simulink model "VDC_2023"  (R2023a)
settings: Solver=FixedStepAuto  StartTime=0.0  StopTime=10.0  RelTol=1e-3
libraries: simulink x4
(part 1 of 2)
settings Model: Creator=no  LastModifiedBy=no
settings OptimizationCC: DefaultParameterBehavior=Inlined
settings RTWCC: Description=INTECRIO Real-Time Target  SystemTargetFile=irt.tlc  TemplateMakefile=irt_default_tmf
settings STFCustomTargetCC: UtilityFuncGeneration=Shared location  ConcurrentExecutionCompliant=off  MatFileLogging=on  UseToolchainInfoCompliant=off  SystemTargetFile=irt.tlc
settings GRTTargetCC: UtilityFuncGeneration=Shared location  ParMdlRefBuildCompliant=off  CompOptLevelCompliant=off  ConcurrentExecutionCompliant=off  CombineOutputUpdateFcns=off  CPPClassGenCompliant=off  GRTInterface=on  UseToolchainInfoCompliant=off  GenerateASAP2=on

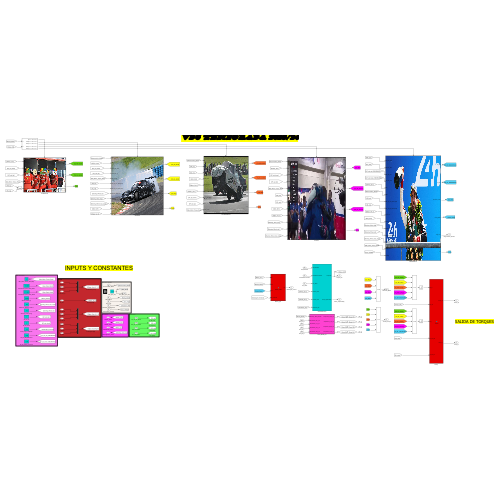
[thumbnail: Simulink's stored preview of the top-level diagram]
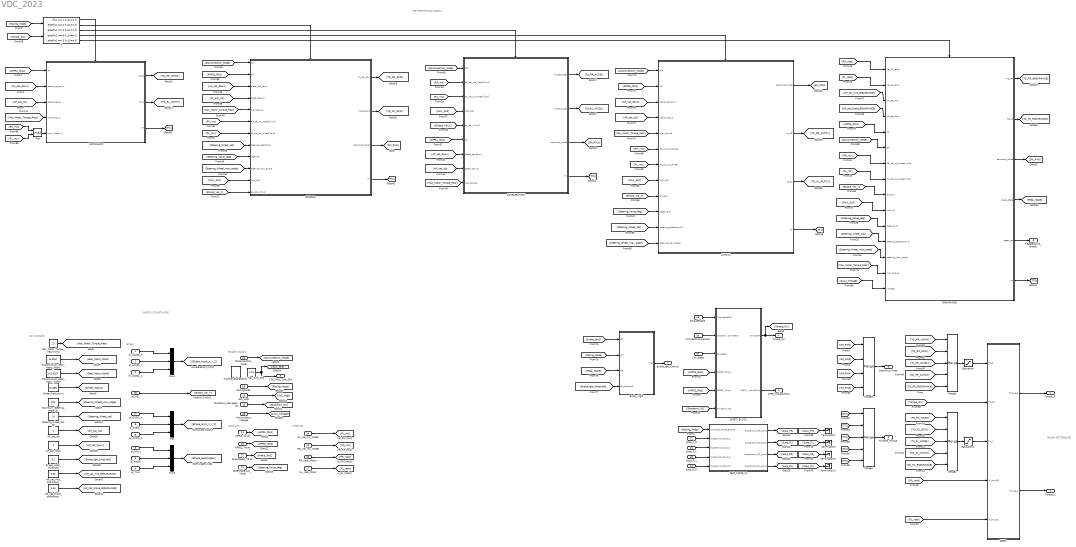
== system VDC_2023 ==
  note: VDC TEMPORADA 2023/24
  note: INPUTS Y CONSTANTES
  note: SALIDA DE TORQUES
  note: Ellipse
  note: Sensorics
  note: Velocities
  note: Car constants
  note: Random Signals
  el_ACCEL_X : Inport
  el_ACCEL_Y : Inport  Port=2
  el_ACCEL_Z : Inport  Port=3
  el_YAW : Inport  Port=4
  el_PITCH : Inport  Port=5
  el_ROLL : Inport  Port=6
  el_GYRO_X : Inport  Port=7
  el_GYRO_Y : Inport  Port=8
  el_GYRO_Z : Inport  Port=9
  APPS2_Value : Inport  Port=10
  APPS1_Value : Inport  Port=11
  BrakePedal_Value : Inport  Port=12
  SteeringSensor_Value : Inport  Port=13
  RL_Vel_ms_Wheel : Inport  Port=14
  RR_Vel_ms_Wheel : Inport  Port=15
  RR_rads_Motor : Inport  Port=16
  RL_rads_Motor : Inport  Port=17
  Accumulator_Voltage : Inport  Port=18
  Shutdown_PackageIntck : Inport  Port=19
  Disconnection_Mode : Inport  Port=20
  Susp_F_L : Inport  Port=21
  Susp_F_R : Inport  Port=22
  Susp_R_L : Inport  Port=23
  Susp_R_R : Inport  Port=24
  TorqueEnable : Inport  Port=25
  CriticalDisconnection : Inport  Port=26
  Car_State : Inport  Port=27
  RacingMode : Inport  Port=28
  SoC_High : Inport  Port=29
  el_VEL : Inport  Port=30
  ACCELERATION : Subsystem
      mask Display: image('flight-simulator-x-4e263b2eefc8e-3478716029.jpg');
  AP_sat_brake_endurance : Constant  Value=0.45
  AP_sat_down : Constant  Value=0
  AP_sat_mid_endurance : Constant  Value=0.55
  AP_sat_up : Constant
  AUTOX1 : Subsystem
      mask Display: image('autox.jpg');
  Brake_Light : MATLAB Function  TreatAsAtomicUnit=on
  Brake_Light_Threshold : Constant  Value=0.2
  ENDURANCE : Subsystem
      mask Display: image('endurance.jpg');
  Function Explanation : simulink/Model-Wide Utilities/DocBlock  DocumentType=Text
      content=|
      | Comparing the speed of the Ellipse and the speed of the Wheels, we can
      | determine the % of deviation between both (which is the slip). With
      | calculations from the Tyres & Performance Department, we know that the
      | maximum optimal slip in a STRAIGHT line is 15%. Therefore (using the Magic
      | Formula), we can determine the maximum X-Force permissible by the Wheels
      | with that % of slip (which is the constant Max_Fx_Tyre, input
      | of Rigid Axle).
      |
      | With that and the radius of the Wheels, we can calculate the maximum
      | Torque for it to stop slipping.
  If : If  NumInputs=2  IfExpression=u1 == 1 & u2 == 1  ElseIfExpressions=u1 == 2 & u2 == 1, u1 == 3 & u2 == 1, u1 == 4 & u2 == 1, u1 == 5 & u2 == 1  ShowElse=off
  Max : MinMax  Function=max  Inputs=2
  Max_Motor_Torque_Rear [Nm] : Constant  Value=27
  Max_Tyre_Slip : Constant  Value=1.15
  Maximum_Steering_angle [º] : Constant  Value=125
  Merge1 : Merge  Inputs=5
  Merge2 : Merge  Inputs=5
  Merge3 : Merge  Inputs=4
  Merge4 : Merge  Inputs=5
  Mux : Mux  Inputs=3
  Mux1 : Mux  Inputs=3
  Mux3 : Mux  Inputs=3
  SAFETY BLOCK : Subsystem
  SKIDPAD : Subsystem
      mask Display: image('MZR_MadMike_Okayama_36_12-4221701208.jpg');
  Safety : MATLAB Function  TreatAsAtomicUnit=on
  Saturation : Saturate  UpperLimit=27  LowerLimit=-27
  Saturation1 : Saturate  UpperLimit=27  LowerLimit=-27
  Steering_wheel_sat [º] : Constant  Value=10
  TEST_MODE_IN : Subsystem  TreatAsAtomicUnit=on
  Terminator{2..3,10..11} (4 alike) : Terminator
  Transmission_Gear_Ratio_MtoW : Constant  Value=11.3257
  Transmission_Gear_Ratio_WtoM : Constant  Value=1/11.3257
  WORKSHOP : Subsystem
      mask Display: image('workshop.jpg');
  Wheel_Radius [m] : Constant  Value=0.2285
  Torque_R : Outport
  Torque_L : Outport  Port=2
  APPS_Implausibility : Outport  Port=3  VectorParamsAs1DForOutWhenUnconnected=off
  Torque_OK : Outport  Port=4  VectorParamsAs1DForOutWhenUnconnected=off
  VDC_Max_Tyre_Slip : Outport  Port=5
  Sensorics_Mode : Outport  Port=6
  BrakeLight_Control : Outport  Port=7  VectorParamsAs1DForOutWhenUnconnected=off
  Regenerative_Enable : Outport  Port=8
  Throttle_Torque : Outport  Port=9
  wires:
  el_PITCH/1 -> Mux3/2
  el_GYRO_Z/1 -> Mux/3
  el_ACCEL_Y/1 -> Mux1/2
  Mux3/1 -> [Ellipse_EulerAngles]
  el_ROLL/1 -> Mux3/1
  Mux1/1 -> [Ellipse_Accel_X_Y_Z]
  el_YAW/1 -> Mux3/3
  el_GYRO_X/1 -> Mux/1
  el_ACCEL_X/1 -> Mux1/1
  Mux/1 -> [Ellipse_Gyro_X_Y_Z]
  el_GYRO_Y/1 -> Mux/2
  el_ACCEL_Z/1 -> Mux1/3
  SteeringSensor_Value/1 -> [Steering_Value_deg]
  APPS1_Value/1 -> [APPS1_0to1]
  BrakePedal_Value/1 -> [Brake_0to1]
  APPS2_Value/1 -> [APPS2_0to1]
  Transmission_Gear_Ratio_MtoW/1 -> [Gear_Ratio_MtoW]
  Transmission_Gear_Ratio_WtoM/1 -> [Gear_Ratio_WtoM]
  Wheel_Radius [m]/1 -> [Wheel_Radius]
  Max_Motor_Torque_Rear [Nm]/1 -> [Max_Motor_Torque_Rear]
  Shutdown_PackageIntck/1 -> [Shutdown_OK]
  Accumulator_Voltage/1 -> [Accu_Voltage]
  Maximum_Steering_angle [º]/1 -> [Steering_Wheel_max_angle]
  Steering_wheel_sat [º]/1 -> [Steering_Wheel_sat]
  Disconnection_Mode/1 -> [Disconnection_Mode]
  TEST_MODE_IN/2(Suspension_FL_N_out) -> [Susp_FL]
  [Racing_Mode] -> TEST_MODE_IN/1(Workshop_Mode_Enable)
  Susp_F_R/1 -> TEST_MODE_IN/2(Suspension_FR_N_in)
  Susp_R_L/1 -> TEST_MODE_IN/4(Suspension_RL_N_in)
  Susp_R_R/1 -> TEST_MODE_IN/5(Suspension_RR_N_in)
  TEST_MODE_IN/3(Suspension_RR_N_out) -> [Susp_RR]
  Susp_F_L/1 -> TEST_MODE_IN/3(Suspension_FL_N_in)
  TEST_MODE_IN/4(Suspension_RL_N_out) -> [Susp_RL]
  TEST_MODE_IN/1(Suspension_FR_N_out) -> [Susp_FR]
  Max_Tyre_Slip/1 -> [MAX_SLR], VDC_Max_Tyre_Slip/1
  CriticalDisconnection/1 -> SAFETY BLOCK/2(CriticalDisconnection)
  TorqueEnable/1 -> SAFETY BLOCK/1(TorqueEnable)
  SAFETY BLOCK/1(TorqueOK) -> Torque_OK/1, [Torque_OK]
  [APPS1_0to1] -> SAFETY BLOCK/4(APPS1_Value)
  SAFETY BLOCK/2(APPS_Implausibility) -> APPS_Implausibility/1
  [APPS2_0to1] -> SAFETY BLOCK/5(APPS2_Value)
  [Shutdown_OK] -> SAFETY BLOCK/6(Shutdown_OK)
  Car_State/1 -> SAFETY BLOCK/3(Car_State)
  AP_sat_up/1 -> [AP_sat_Up]
  AP_sat_down/1 -> [AP_sat_down]
  [Susp_FL] -> Terminator3/1
  [Susp_RL] -> Terminator11/1
  [Susp_RR] -> Terminator10/1
  [Susp_FR] -> Terminator2/1
  [Tq_RR_ACCEL] -> Merge2/3
  [TQ_RR_AUTOX] -> Merge2/4
  [TQ_RR_WORK] -> Merge2/1
  [TQ_RR_SKID] -> Merge2/2
  RacingMode/1 -> [Racing_Mode]
  [APPS1_0to1] -> WORKSHOP/1(AP)
  [AP_sat_down] -> WORKSHOP/2(pedal_sat_down)
  [AP_sat_Up] -> WORKSHOP/3(pedal_sat_up)
  [Max_Motor_Torque_Rear] -> WORKSHOP/4(max_torque)
  [TQ_RR_ENDURANCE] -> Merge2/5
  [TQ_RL_ENDURANCE] -> Merge1/5
  [TQ_RL_SKID] -> Merge1/2
  [TQ_RL_AUTOX] -> Merge1/4
  [Tq_RL_ACCEL] -> Merge1/3
  [TQ_RL_WORK] -> Merge1/1
  WORKSHOP/1(TQ_R) -> [TQ_RR_WORK]
  WORKSHOP/2(TQ_L) -> [TQ_RL_WORK]
  ENDURANCE/2(TQ_RL) -> [TQ_RL_ENDURANCE]
  ENDURANCE/1(TQ_RR) -> [TQ_RR_ENDURANCE]
  [Racing_Mode] -> If/1
  If/1 -> WORKSHOP/Action
  If/2 -> SKIDPAD/Action
  If/3 -> ACCELERATION/Action
  If/4 -> AUTOX1/Action
  If/5 -> ENDURANCE/Action
  [MAX_SLR] -> ENDURANCE/10(max_slr)
  [Disconnection_Mode] -> ENDURANCE/6(DM)
  RL_rads_Motor/1 -> [RL_rads]
  RR_rads_Motor/1 -> [RR_rads]
  RR_Vel_ms_Wheel/1 -> [RR_ms]
  RL_Vel_ms_Wheel/1 -> [RL_ms]
  [RR_rads] -> ENDURANCE/1(Vel_RR_rad/s)
  [RL_rads] -> ENDURANCE/2(Vel_RL_rad/s)
  [RR_ms] -> ENDURANCE/7(RR_Vel_ms_Wheel [m/s])
  [RL_ms] -> ENDURANCE/8(RL_Vel_ms_Wheel [m/s])
  [Steering_Wheel_sat] -> ENDURANCE/12(steering_deadzone (º))
  [Steering_Value_deg] -> ENDURANCE/11(steering (º))
  [Steering_Wheel_max_angle] -> ENDURANCE/13(steering_max_angle)
  [APPS1_0to1] -> ENDURANCE/5(AP)
  SoC_High/1 -> [SoC_High]
  ACCELERATION/1(Tq_RR_accel) -> [Tq_RR_ACCEL]
  ACCELERATION/2(Tq_RL_accel) -> [Tq_RL_ACCEL]
  SKIDPAD/1(Tq_RR_Skid) -> [TQ_RR_SKID]
  SKIDPAD/2(Tq_RL_Skid) -> [TQ_RL_SKID]
  [Disconnection_Mode] -> SKIDPAD/1(DM)
  [Disconnection_Mode] -> ACCELERATION/1(DM)
  [RR_ms] -> SKIDPAD/6(RR_Vel_ms_Wheel [m/s])
  [RL_ms] -> SKIDPAD/7(RL_Vel_ms_Wheel [m/s])
  [RL_ms] -> ACCELERATION/3(RL_Vel_ms_Wheel [m/s])
  [RR_ms] -> ACCELERATION/2(RR_Vel_ms_Wheel [m/s])
  [APPS1_0to1] -> SKIDPAD/2(AP)
  [Steering_Value_deg] -> SKIDPAD/9(steering)
  [APPS1_0to1] -> ACCELERATION/6(AP)
  [AP_sat_down] -> SKIDPAD/3(pedal_sat_down)
  [AP_sat_Up] -> SKIDPAD/4(pedal_sat_up)
  [AP_sat_down] -> ACCELERATION/7(pedal_sat_down)
  [AP_sat_Up] -> ACCELERATION/8(pedal_sat_up)
  [Max_Motor_Torque_Rear] -> SKIDPAD/5(max_torque)
  [Max_Motor_Torque_Rear] -> ACCELERATION/9(max_torque)
  [MAX_SLR] -> SKIDPAD/11(MAX_SLR)
  [Steering_Wheel_sat] -> SKIDPAD/8(steering_deadzone)
  [Steering_Wheel_max_angle] -> SKIDPAD/10(steering_max_angle)
  [MAX_SLR] -> ACCELERATION/4(MAX_SLR)
  [Torque_OK] -> If/2
  Merge3/1 -> Sensorics_Mode/1
  [SM_RM2] -> Merge3/1
  [SM_RM4] -> Merge3/3
  [SM_RM5] -> Merge3/4
  [SM_RM3] -> Merge3/2
  SKIDPAD/3(sensorics_mode) -> [SM_RM2]
  ACCELERATION/3(sensorics_mode) -> [SM_RM3]
  ENDURANCE/3(sensorics_mode) -> [SM_RM5]
  AUTOX1/1(sensorics_mode) -> [SM_RM4]
  AUTOX1/2(tq_RR) -> [TQ_RR_AUTOX]
  AUTOX1/3(tq_RL) -> [TQ_RL_AUTOX]
  [Steering_Wheel_max_angle] -> AUTOX1/12(steering_max_angle)
  [Steering_Value_deg] -> AUTOX1/10(steering (º))
  [Steering_Wheel_sat] -> AUTOX1/11(steering_deadzone (º))
  [MAX_SLR] -> AUTOX1/8(MAX_SLR)
  [RR_ms] -> AUTOX1/6(RR_vel_ms_Wheel)
  [RL_ms] -> AUTOX1/7(RL_vel_ms_Wheel)
  [Max_Motor_Torque_Rear] -> AUTOX1/5(max_torque)
  [Disconnection_Mode] -> AUTOX1/1(DM)
  [APPS1_0to1] -> AUTOX1/2(AP)
  [AP_sat_down] -> AUTOX1/3(pedal_sat_down)
  [AP_sat_Up] -> AUTOX1/4(pedal_sat_up)
  ENDURANCE/4(Pedal_State) -> [Pedal_State]
  Brake_Light_Threshold/1 -> [BrakeLight_threshold]
  Brake_Light/1(BL) -> BrakeLight_Control/1
  [Brake_0to1] -> Brake_Light/1(BP)
  [Racing_Mode] -> Brake_Light/2(RM)
  [BrakeLight_threshold] -> Brake_Light/4(BL_threshold)
  [Pedal_State] -> Brake_Light/3(PS)
  [Max_Motor_Torque_Rear] -> ENDURANCE/14(max_torque)
  Merge2/1 -> Saturation/1
  Saturation/1 -> Safety/1(Tq_R)
  Merge1/1 -> Saturation1/1
  ENDURANCE/5(regen_en) -> Regenerative_Enable/1
  [Accu_Voltage] -> ENDURANCE/15(voltage)
  WORKSHOP/3(TT) -> [TT1]
  SKIDPAD/4(TT) -> [TT2]
  ACCELERATION/4(TT) -> [TT3]
  AUTOX1/4(TT) -> [TT4]
  ENDURANCE/6(TT) -> [TT5]
  Merge4/1 -> Throttle_Torque/1
  [TT1] -> Merge4/1
  [TT2] -> Merge4/2
  [TT3] -> Merge4/3
  [TT4] -> Merge4/4
  [TT5] -> Merge4/5
  Saturation1/1 -> Safety/3(Tq_L)
  Safety/2(Torque_L) -> Torque_L/1
  Safety/1(Torque_R) -> Torque_R/1
  [Torque_OK] -> Safety/2(Tq_OK)
  [RR_rads] -> Safety/4(W_mot_RR)
  [RL_rads] -> Safety/5(W_mot_RL)
  Max/1 -> WORKSHOP/5(max_wheel_w)
  [RR_ms] -> Max/1
  [RL_ms] -> Max/2
  AP_sat_mid_endurance/1 -> [AP_sat_mid_ENDURANCE]
  AP_sat_brake_endurance/1 -> [AP_sat_brake_ENDURANCE]
  [AP_sat_mid_ENDURANCE] -> ENDURANCE/3(AP_sat_mid)
  [AP_sat_brake_ENDURANCE] -> ENDURANCE/4(AP_sat_down)
  el_VEL/1 -> [Ellipse_Vel_X]
  [Ellipse_Vel_X] -> SKIDPAD/12(el_Vel_X [m/s])
  [Ellipse_Vel_X] -> ACCELERATION/5(el_Vel_X [m/s])
  [Ellipse_Vel_X] -> AUTOX1/9(el_vel_x)
  [Ellipse_Vel_X] -> ENDURANCE/9(el_Vel_X)

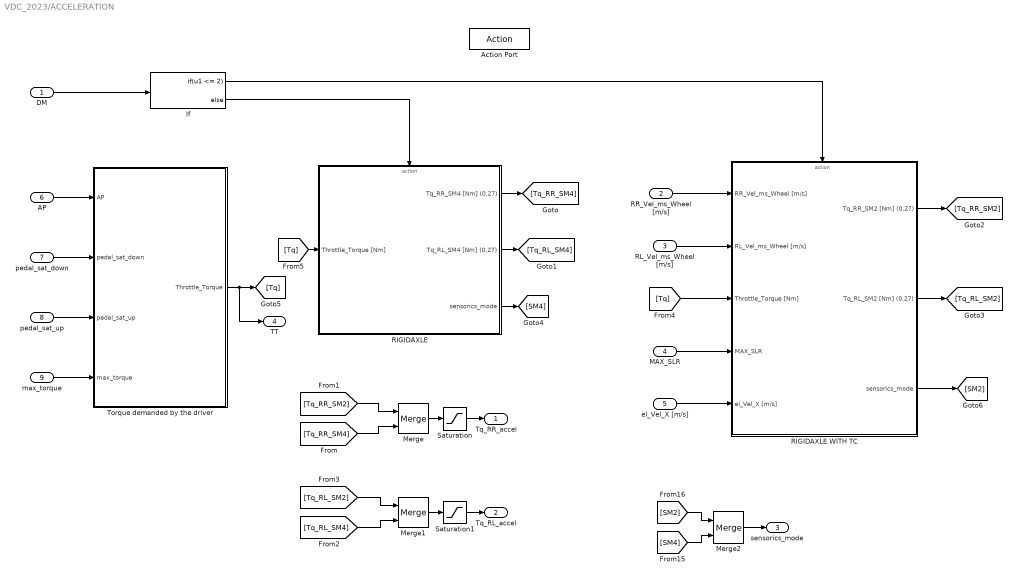
== system VDC_2023/ACCELERATION ==
  DM : Inport
  RR_Vel_ms_Wheel [m/s] : Inport  Port=2
  RL_Vel_ms_Wheel [m/s] : Inport  Port=3
  MAX_SLR : Inport  Port=4
  el_Vel_X [m/s] : Inport  Port=5
  AP : Inport  Port=6
  pedal_sat_down : Inport  Port=7
  pedal_sat_up : Inport  Port=8
  max_torque : Inport  Port=9
  Action Port : ActionPort  ActionPortLabel=elseif( u1 == 3 & u2 == 1)
  If : If  IfExpression=u1 <= 2
  Merge : Merge
  Merge1 : Merge
  Merge2 : Merge
  RIGIDAXLE : Subsystem
  RIGIDAXLE WITH TC : Subsystem
  Saturation : Saturate  UpperLimit=27  LowerLimit=0
  Saturation1 : Saturate  UpperLimit=27  LowerLimit=0
  Torque demanded by the driver : MATLAB Function  TreatAsAtomicUnit=on
  Tq_RR_accel : Outport
  Tq_RL_accel : Outport  Port=2
  sensorics_mode : Outport  Port=3
  TT : Outport  Port=4
  wires:
  DM/1 -> If/1
  If/2 -> RIGIDAXLE/Action
  el_Vel_X [m/s]/1 -> RIGIDAXLE WITH TC/5(el_Vel_X [m/s])
  MAX_SLR/1 -> RIGIDAXLE WITH TC/4(MAX_SLR)
  RL_Vel_ms_Wheel [m/s]/1 -> RIGIDAXLE WITH TC/2(RL_Vel_ms_Wheel [m/s])
  RR_Vel_ms_Wheel [m/s]/1 -> RIGIDAXLE WITH TC/1(RR_Vel_ms_Wheel [m/s])
  AP/1 -> Torque demanded by the driver/1(AP)
  pedal_sat_down/1 -> Torque demanded by the driver/2(pedal_sat_down)
  pedal_sat_up/1 -> Torque demanded by the driver/3(pedal_sat_up)
  max_torque/1 -> Torque demanded by the driver/4(max_torque)
  RIGIDAXLE/1(Tq_RR_SM4 [Nm] (0,27)) -> [Tq_RR_SM4]
  RIGIDAXLE/2(Tq_RL_SM4 [Nm] (0,27)) -> [Tq_RL_SM4]
  RIGIDAXLE WITH TC/2(Tq_RL_SM2 [Nm] (0,27)) -> [Tq_RL_SM2]
  RIGIDAXLE WITH TC/1(Tq_RR_SM2 [Nm] (0,27)) -> [Tq_RR_SM2]
  [Tq_RR_SM4] -> Merge/2
  [Tq_RR_SM2] -> Merge/1
  [Tq_RL_SM4] -> Merge1/2
  [Tq_RL_SM2] -> Merge1/1
  Merge2/1 -> sensorics_mode/1
  [SM4] -> Merge2/2
  [SM2] -> Merge2/1
  RIGIDAXLE/3(sensorics_mode) -> [SM4]
  Torque demanded by the driver/1(Throttle_Torque) -> TT/1, [Tq]
  [Tq] -> RIGIDAXLE WITH TC/3(Throttle_Torque [Nm])
  [Tq] -> RIGIDAXLE/1(Throttle_Torque [Nm])
  RIGIDAXLE WITH TC/3(sensorics_mode) -> [SM2]
  If/1 -> RIGIDAXLE WITH TC/Action
  Merge/1 -> Saturation/1
  Saturation/1 -> Tq_RR_accel/1
  Merge1/1 -> Saturation1/1
  Saturation1/1 -> Tq_RL_accel/1

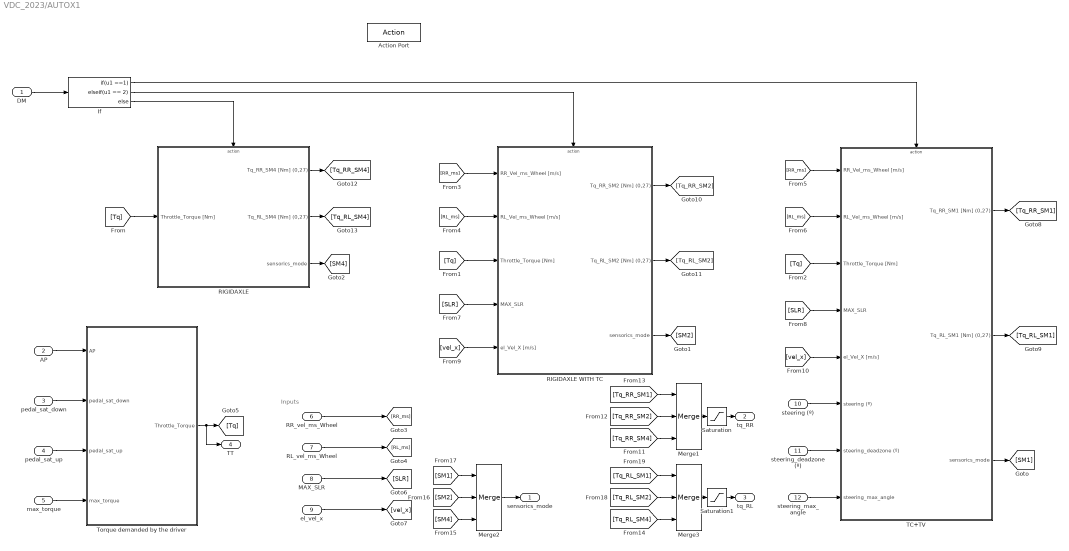
== system VDC_2023/AUTOX1 ==
  note: Inputs
  DM : Inport
  AP : Inport  Port=2
  pedal_sat_down : Inport  Port=3
  pedal_sat_up : Inport  Port=4
  max_torque : Inport  Port=5
  RR_vel_ms_Wheel : Inport  Port=6
  RL_vel_ms_Wheel : Inport  Port=7
  MAX_SLR : Inport  Port=8
  el_vel_x : Inport  Port=9
  steering (º) : Inport  Port=10
  steering_deadzone (º) : Inport  Port=11
  steering_max_angle : Inport  Port=12
  Action Port : ActionPort  ActionPortLabel=elseif( u1 == 4 & u2 == 1)
  If : If  IfExpression=u1 ==1  ElseIfExpressions=u1 == 2
  Merge1 : Merge  Inputs=3
  Merge2 : Merge  Inputs=3
  Merge3 : Merge  Inputs=3
  RIGIDAXLE : Subsystem
  RIGIDAXLE WITH TC : Subsystem
  Saturation : Saturate  UpperLimit=27  LowerLimit=0
  Saturation1 : Saturate  UpperLimit=27  LowerLimit=0
  TC+TV : Subsystem
  Torque demanded by the driver : MATLAB Function  TreatAsAtomicUnit=on
  sensorics_mode : Outport
  tq_RR : Outport  Port=2
  tq_RL : Outport  Port=3
  TT : Outport  Port=4
  wires:
  RIGIDAXLE WITH TC/3(sensorics_mode) -> [SM2]
  TC+TV/3(sensorics_mode) -> [SM1]
  RIGIDAXLE/3(sensorics_mode) -> [SM4]
  [SM2] -> Merge2/2
  [SM4] -> Merge2/3
  Merge2/1 -> sensorics_mode/1
  [SM1] -> Merge2/1
  If/1 -> TC+TV/Action
  If/2 -> RIGIDAXLE WITH TC/Action
  If/3 -> RIGIDAXLE/Action
  DM/1 -> If/1
  pedal_sat_down/1 -> Torque demanded by the driver/2(pedal_sat_down)
  Torque demanded by the driver/1(Throttle_Torque) -> TT/1, [Tq]
  max_torque/1 -> Torque demanded by the driver/4(max_torque)
  pedal_sat_up/1 -> Torque demanded by the driver/3(pedal_sat_up)
  AP/1 -> Torque demanded by the driver/1(AP)
  [Tq] -> RIGIDAXLE/1(Throttle_Torque [Nm])
  [Tq] -> RIGIDAXLE WITH TC/3(Throttle_Torque [Nm])
  [Tq] -> TC+TV/3(Throttle_Torque [Nm])
  RR_vel_ms_Wheel/1 -> [RR_ms]
  RL_vel_ms_Wheel/1 -> [RL_ms]
  [RR_ms] -> RIGIDAXLE WITH TC/1(RR_Vel_ms_Wheel [m/s])
  [RL_ms] -> RIGIDAXLE WITH TC/2(RL_Vel_ms_Wheel [m/s])
  [RR_ms] -> TC+TV/1(RR_Vel_ms_Wheel [m/s])
  [RL_ms] -> TC+TV/2(RL_Vel_ms_Wheel [m/s])
  MAX_SLR/1 -> [SLR]
  el_vel_x/1 -> [vel_x]
  [SLR] -> RIGIDAXLE WITH TC/4(MAX_SLR)
  [SLR] -> TC+TV/4(MAX_SLR)
  [vel_x] -> RIGIDAXLE WITH TC/5(el_Vel_X [m/s])
  [vel_x] -> TC+TV/5(el_Vel_X [m/s])
  steering (º)/1 -> TC+TV/6(steering (º))
  steering_deadzone (º)/1 -> TC+TV/7(steering_deadzone (º))
  steering_max_angle/1 -> TC+TV/8(steering_max_angle)
  [Tq_RR_SM4] -> Merge1/3
  [Tq_RR_SM1] -> Merge1/1
  [Tq_RR_SM2] -> Merge1/2
  [Tq_RL_SM4] -> Merge3/3
  [Tq_RL_SM1] -> Merge3/1
  [Tq_RL_SM2] -> Merge3/2
  TC+TV/1(Tq_RR_SM1 [Nm] (0,27)) -> [Tq_RR_SM1]
  TC+TV/2(Tq_RL_SM1 [Nm] (0,27)) -> [Tq_RL_SM1]
  RIGIDAXLE WITH TC/1(Tq_RR_SM2 [Nm] (0,27)) -> [Tq_RR_SM2]
  RIGIDAXLE WITH TC/2(Tq_RL_SM2 [Nm] (0,27)) -> [Tq_RL_SM2]
  RIGIDAXLE/2(Tq_RL_SM4 [Nm] (0,27)) -> [Tq_RL_SM4]
  RIGIDAXLE/1(Tq_RR_SM4 [Nm] (0,27)) -> [Tq_RR_SM4]
  Merge1/1 -> Saturation/1
  Saturation/1 -> tq_RR/1
  Merge3/1 -> Saturation1/1
  Saturation1/1 -> tq_RL/1

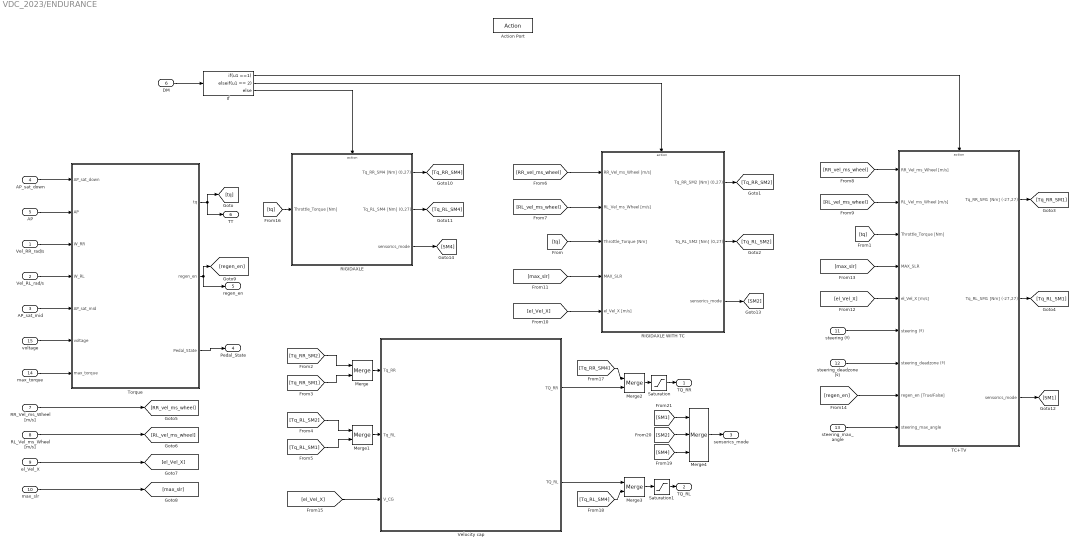
== system VDC_2023/ENDURANCE ==
  Vel_RR_rad/s : Inport
  Vel_RL_rad/s : Inport  Port=2
  AP_sat_mid : Inport  Port=3
  AP_sat_down : Inport  Port=4
  AP : Inport  Port=5
  DM : Inport  Port=6
  RR_Vel_ms_Wheel [m/s] : Inport  Port=7
  RL_Vel_ms_Wheel [m/s] : Inport  Port=8
  el_Vel_X : Inport  Port=9
  max_slr : Inport  Port=10
  steering (º) : Inport  Port=11
  steering_deadzone (º) : Inport  Port=12
  steering_max_angle : Inport  Port=13
  max_torque : Inport  Port=14
  voltage : Inport  Port=15
  Action Port : ActionPort  ActionPortLabel=elseif( u1 == 5 & u2 == 1)
  If : If  IfExpression=u1 ==1  ElseIfExpressions=u1 == 2
  Merge{,1..3} (4 alike) : Merge
  Merge4 : Merge  Inputs=3
  RIGIDAXLE : Subsystem
  RIGIDAXLE WITH TC : Subsystem
  Saturation : Saturate  UpperLimit=27  LowerLimit=-27
  Saturation1 : Saturate  UpperLimit=27  LowerLimit=-27
  TC+TV : Subsystem
  Torque : Subsystem
  Velocity cap : Subsystem
      mask Display: image('iStock-173100947-1675497781.jpg');
  TQ_RR : Outport
  TQ_RL : Outport  Port=2
  sensorics_mode : Outport  Port=3
  Pedal_State : Outport  Port=4
  regen_en : Outport  Port=5
  TT : Outport  Port=6
  wires:
  [tq] -> RIGIDAXLE WITH TC/3(Throttle_Torque [Nm])
  [tq] -> TC+TV/3(Throttle_Torque [Nm])
  RIGIDAXLE WITH TC/1(Tq_RR_SM2 [Nm] (0,27)) -> [Tq_RR_SM2]
  RIGIDAXLE WITH TC/2(Tq_RL_SM2 [Nm] (0,27)) -> [Tq_RL_SM2]
  [Tq_RR_SM2] -> Merge/1
  [Tq_RR_SM1] -> Merge/2
  [Tq_RL_SM2] -> Merge1/1
  [Tq_RL_SM1] -> Merge1/2
  TC+TV/1(Tq_RR_SM1 [Nm] (-27,27)) -> [Tq_RR_SM1]
  TC+TV/2(Tq_RL_SM1 [Nm] (-27,27)) -> [Tq_RL_SM1]
  Merge/1 -> Velocity cap/1(Tq_RR)
  Merge1/1 -> Velocity cap/2(Tq_RL)
  Vel_RR_rad/s/1 -> Torque/3(W_RR)
  Vel_RL_rad/s/1 -> Torque/4(W_RL)
  AP_sat_mid/1 -> Torque/5(AP_sat_mid)
  AP_sat_down/1 -> Torque/1(AP_sat_down)
  AP/1 -> Torque/2(AP)
  DM/1 -> If/1
  RR_Vel_ms_Wheel [m/s]/1 -> [RR_vel_ms_wheel]
  [RR_vel_ms_wheel] -> RIGIDAXLE WITH TC/1(RR_Vel_ms_Wheel [m/s])
  RL_Vel_ms_Wheel [m/s]/1 -> [RL_vel_ms_wheel]
  [RL_vel_ms_wheel] -> RIGIDAXLE WITH TC/2(RL_Vel_ms_Wheel [m/s])
  [RR_vel_ms_wheel] -> TC+TV/1(RR_Vel_ms_Wheel [m/s])
  [RL_vel_ms_wheel] -> TC+TV/2(RL_Vel_ms_Wheel [m/s])
  el_Vel_X/1 -> [el_Vel_X]
  [el_Vel_X] -> RIGIDAXLE WITH TC/5(el_Vel_X [m/s])
  max_slr/1 -> [max_slr]
  [max_slr] -> RIGIDAXLE WITH TC/4(MAX_SLR)
  [el_Vel_X] -> TC+TV/5(el_Vel_X [m/s])
  [max_slr] -> TC+TV/4(MAX_SLR)
  steering (º)/1 -> TC+TV/6(steering (º))
  steering_deadzone (º)/1 -> TC+TV/7(steering_deadzone (º))
  Torque/2(regen_en) -> [regen_en], regen_en/1
  [regen_en] -> TC+TV/8(regen_en [True/False])
  steering_max_angle/1 -> TC+TV/9(steering_max_angle)
  [el_Vel_X] -> Velocity cap/3(V_CG)
  If/2 -> RIGIDAXLE WITH TC/Action
  If/1 -> TC+TV/Action
  [tq] -> RIGIDAXLE/1(Throttle_Torque [Nm])
  RIGIDAXLE/1(Tq_RR_SM4 [Nm] (0,27)) -> [Tq_RR_SM4]
  RIGIDAXLE/2(Tq_RL_SM4 [Nm] (0,27)) -> [Tq_RL_SM4]
  Velocity cap/1(TQ_RR) -> Merge2/2
  [Tq_RR_SM4] -> Merge2/1
  Velocity cap/2(TQ_RL) -> Merge3/1
  [Tq_RL_SM4] -> Merge3/2
  If/3 -> RIGIDAXLE/Action
  [SM1] -> Merge4/1
  Merge4/1 -> sensorics_mode/1
  [SM4] -> Merge4/3
  [SM2] -> Merge4/2
  TC+TV/3(sensorics_mode) -> [SM1]
  RIGIDAXLE WITH TC/3(sensorics_mode) -> [SM2]
  RIGIDAXLE/3(sensorics_mode) -> [SM4]
  Torque/3(Pedal_State) -> Pedal_State/1
  max_torque/1 -> Torque/7(max_torque)
  voltage/1 -> Torque/6(voltage)
  Merge2/1 -> Saturation/1
  Saturation/1 -> TQ_RR/1
  Merge3/1 -> Saturation1/1
  Saturation1/1 -> TQ_RL/1
  Torque/1(tq) -> [tq], TT/1

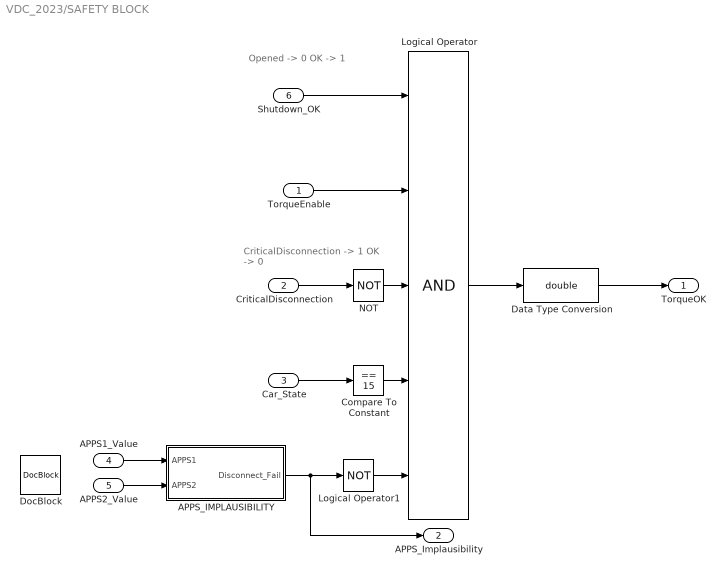
== system VDC_2023/SAFETY BLOCK ==
  note: CriticalDisconnection -> 1
      | OK -> 0
  note: Opened -> 0
      | OK -> 1
  TorqueEnable : Inport
  CriticalDisconnection : Inport  Port=2
  Car_State : Inport  Port=3
  APPS1_Value : Inport  Port=4
  APPS2_Value : Inport  Port=5
  Shutdown_OK : Inport  Port=6
  APPS_IMPLAUSIBILITY : Subsystem
  Compare To Constant : simulink/Logic and Bit Operations/Compare To Constant  relop===  const=15  OutDataTypeStr=boolean
  Data Type Conversion : DataTypeConversion  OutDataTypeStr=double  SaturateOnIntegerOverflow=off  RndMeth=Floor
  DocBlock : simulink/Model-Wide Utilities/DocBlock  DocumentType=Text
      content=|
      | Formula Student Rules 2024 -> T11.8.8
      |     If an implausibility occurs between the values of the APPSs and
      |     persists for more than 100 ms:
      |     • [EV ONLY] The power to the motor(s) must be immediately shut down
      |     completely. It is not necessary to completely deactivate the TS, the
      |     motor controller(s) shutting down the power to the motor(s) is
      |     sufficient.
      |
      | The 'Number_of_Periods' constant, if there's an Implausability, outputs the error X
      | periods (100ms) after the Implausibility happened (25ms * X = 100ms).
  Logical Operator : Logic  Inputs=5  OutDataTypeStr=boolean
  Logical Operator1 : Logic  Operator=NOT  IconShape=distinctive  AllPortsSameDT=off  OutDataTypeStr=boolean
  NOT : Logic  Operator=NOT  IconShape=distinctive  AllPortsSameDT=off  OutDataTypeStr=boolean
  TorqueOK : Outport  VectorParamsAs1DForOutWhenUnconnected=off
  APPS_Implausibility : Outport  Port=2  VectorParamsAs1DForOutWhenUnconnected=off
  wires:
  Logical Operator/1 -> Data Type Conversion/1
  Car_State/1 -> Compare To Constant/1
  NOT/1 -> Logical Operator/3
  CriticalDisconnection/1 -> NOT/1
  TorqueEnable/1 -> Logical Operator/2
  APPS2_Value/1 -> APPS_IMPLAUSIBILITY/2(APPS2)
  APPS1_Value/1 -> APPS_IMPLAUSIBILITY/1(APPS1)
  APPS_IMPLAUSIBILITY/1(Disconnect_Fail) -> APPS_Implausibility/1, Logical Operator1/1
  Compare To Constant/1 -> Logical Operator/4
  Shutdown_OK/1 -> Logical Operator/1
  Logical Operator1/1 -> Logical Operator/5
  Data Type Conversion/1 -> TorqueOK/1

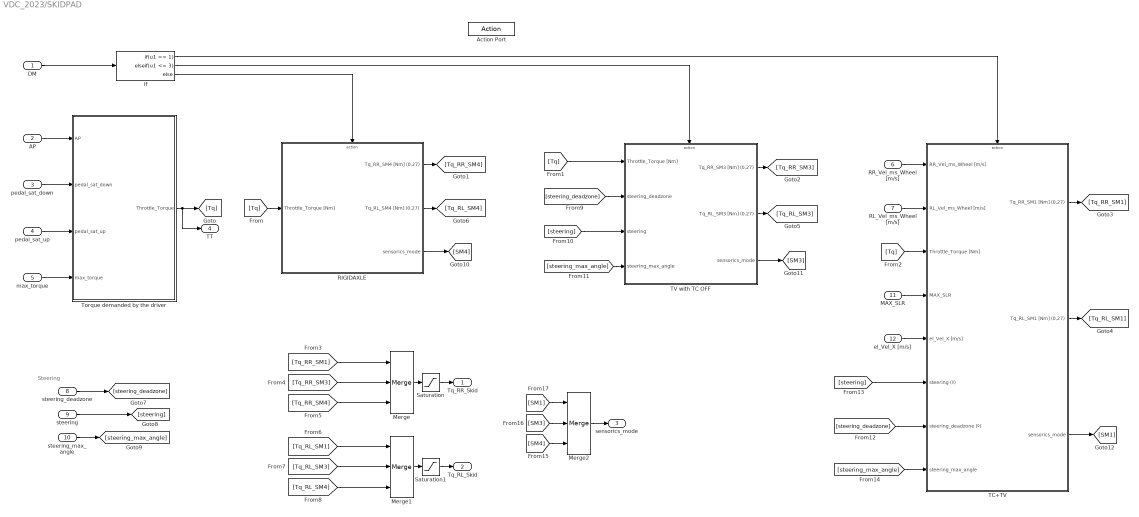
== system VDC_2023/SKIDPAD ==
  note: Steering
  DM : Inport
  AP : Inport  Port=2
  pedal_sat_down : Inport  Port=3
  pedal_sat_up : Inport  Port=4
  max_torque : Inport  Port=5
  RR_Vel_ms_Wheel [m/s] : Inport  Port=6
  RL_Vel_ms_Wheel [m/s] : Inport  Port=7
  steering_deadzone : Inport  Port=8
  steering : Inport  Port=9
  steering_max_angle : Inport  Port=10
  MAX_SLR : Inport  Port=11
  el_Vel_X [m/s] : Inport  Port=12
  Action Port : ActionPort  ActionPortLabel=elseif(u1 == 2 & u2 == 1)
  If : If  IfExpression=u1 == 1  ElseIfExpressions=u1 <= 3
  Merge : Merge  Inputs=3
  Merge1 : Merge  Inputs=3
  Merge2 : Merge  Inputs=3
  RIGIDAXLE : Subsystem
  Saturation : Saturate  UpperLimit=27  LowerLimit=0
  Saturation1 : Saturate  UpperLimit=27  LowerLimit=0
  TC+TV : Subsystem
  "TV with TC OFF " : Subsystem
  Torque demanded by the driver : MATLAB Function  TreatAsAtomicUnit=on
  Tq_RR_Skid : Outport
  Tq_RL_Skid : Outport  Port=2
  sensorics_mode : Outport  Port=3
  TT : Outport  Port=4
  wires:
  DM/1 -> If/1
  If/1 -> TC+TV/Action
  If/3 -> RIGIDAXLE/Action
  pedal_sat_up/1 -> Torque demanded by the driver/3(pedal_sat_up)
  pedal_sat_down/1 -> Torque demanded by the driver/2(pedal_sat_down)
  max_torque/1 -> Torque demanded by the driver/4(max_torque)
  AP/1 -> Torque demanded by the driver/1(AP)
  Torque demanded by the driver/1(Throttle_Torque) -> TT/1, [Tq]
  [Tq] -> RIGIDAXLE/1(Throttle_Torque [Nm])
  [Tq] -> "TV with TC OFF "/1(Throttle_Torque [Nm])
  [Tq] -> TC+TV/3(Throttle_Torque [Nm])
  RR_Vel_ms_Wheel [m/s]/1 -> TC+TV/1(RR_Vel_ms_Wheel [m/s])
  RL_Vel_ms_Wheel [m/s]/1 -> TC+TV/2(RL_Vel_ms_Wheel [m/s])
  [Tq_RR_SM1] -> Merge/1
  [Tq_RR_SM3] -> Merge/2
  [Tq_RR_SM4] -> Merge/3
  RIGIDAXLE/1(Tq_RR_SM4 [Nm] (0,27)) -> [Tq_RR_SM4]
  "TV with TC OFF "/1(Tq_RR_SM3 [Nm] (0,27)) -> [Tq_RR_SM3]
  TC+TV/1(Tq_RR_SM1 [Nm] (0,27)) -> [Tq_RR_SM1]
  [Tq_RL_SM1] -> Merge1/1
  [Tq_RL_SM3] -> Merge1/2
  [Tq_RL_SM4] -> Merge1/3
  TC+TV/2(Tq_RL_SM1 [Nm] (0,27)) -> [Tq_RL_SM1]
  "TV with TC OFF "/2(Tq_RL_SM3 [Nm] (0,27)) -> [Tq_RL_SM3]
  RIGIDAXLE/2(Tq_RL_SM4 [Nm] (0,27)) -> [Tq_RL_SM4]
  steering_deadzone/1 -> [steering_deadzone]
  steering/1 -> [steering]
  steering_max_angle/1 -> [steering_max_angle]
  [steering_deadzone] -> "TV with TC OFF "/2(steering_deadzone)
  [steering] -> "TV with TC OFF "/3(steering)
  [steering_max_angle] -> "TV with TC OFF "/4(steering_max_angle)
  el_Vel_X [m/s]/1 -> TC+TV/5(el_Vel_X [m/s])
  MAX_SLR/1 -> TC+TV/4(MAX_SLR)
  [steering_max_angle] -> TC+TV/8(steering_max_angle)
  [steering] -> TC+TV/6(steering (º))
  [steering_deadzone] -> TC+TV/7(steering_deadzone (º))
  Merge2/1 -> sensorics_mode/1
  RIGIDAXLE/3(sensorics_mode) -> [SM4]
  TC+TV/3(sensorics_mode) -> [SM1]
  "TV with TC OFF "/3(sensorics_mode) -> [SM3]
  [SM4] -> Merge2/3
  [SM3] -> Merge2/2
  [SM1] -> Merge2/1
  If/2 -> "TV with TC OFF "/Action
  Merge/1 -> Saturation/1
  Saturation/1 -> Tq_RR_Skid/1
  Merge1/1 -> Saturation1/1
  Saturation1/1 -> Tq_RL_Skid/1

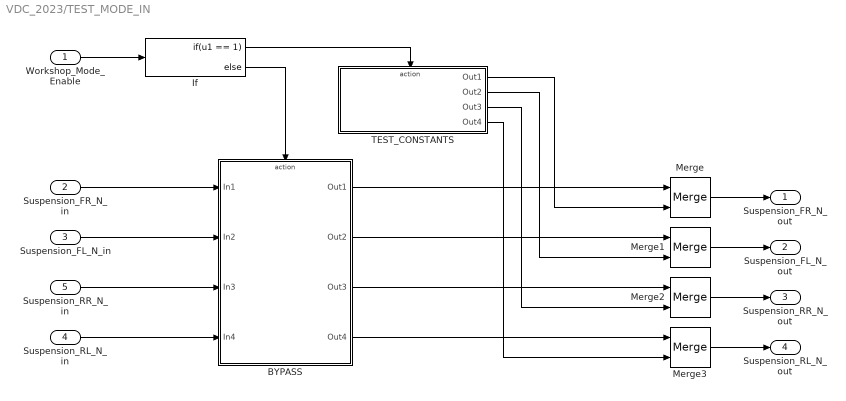
== system VDC_2023/TEST_MODE_IN ==
  Workshop_Mode_Enable : Inport
  Suspension_FR_N_in : Inport  Port=2
  Suspension_FL_N_in : Inport  Port=3
  Suspension_RL_N_in : Inport  Port=4
  Suspension_RR_N_in : Inport  Port=5
  BYPASS : Subsystem  TreatAsAtomicUnit=on
  If : If  IfExpression=u1 == 1
  Merge{,1..3} (4 alike) : Merge
  TEST_CONSTANTS : Subsystem  TreatAsAtomicUnit=on
  Suspension_FR_N_out : Outport  VectorParamsAs1DForOutWhenUnconnected=off
  Suspension_FL_N_out : Outport  Port=2  VectorParamsAs1DForOutWhenUnconnected=off
  Suspension_RR_N_out : Outport  Port=3  VectorParamsAs1DForOutWhenUnconnected=off
  Suspension_RL_N_out : Outport  Port=4  VectorParamsAs1DForOutWhenUnconnected=off
  wires:
  Suspension_FR_N_in/1 -> BYPASS/1(In1)
  Suspension_FL_N_in/1 -> BYPASS/2(In2)
  Suspension_RR_N_in/1 -> BYPASS/3(In3)
  Suspension_RL_N_in/1 -> BYPASS/4(In4)
  Merge/1 -> Suspension_FR_N_out/1
  Merge1/1 -> Suspension_FL_N_out/1
  Merge2/1 -> Suspension_RR_N_out/1
  Merge3/1 -> Suspension_RL_N_out/1
  BYPASS/1(Out1) -> Merge/1
  BYPASS/2(Out2) -> Merge1/1
  BYPASS/3(Out3) -> Merge2/1
  BYPASS/4(Out4) -> Merge3/1
  Workshop_Mode_Enable/1 -> If/1
  If/2 -> BYPASS/Action
  If/1 -> TEST_CONSTANTS/Action
  TEST_CONSTANTS/4(Out4) -> Merge3/2
  TEST_CONSTANTS/3(Out3) -> Merge2/2
  TEST_CONSTANTS/2(Out2) -> Merge1/2
  TEST_CONSTANTS/1(Out1) -> Merge/2

== system VDC_2023/WORKSHOP ==
  AP : Inport
  pedal_sat_down : Inport  Port=2
  pedal_sat_up : Inport  Port=3
  max_torque : Inport  Port=4
  max_wheel_w : Inport  Port=5
  Action Port : ActionPort  ActionPortLabel=if(u1 == 1 & u2 == 1)
  Saturation : Saturate  UpperLimit=3  LowerLimit=0
  Torque demanded by the driver : MATLAB Function  TreatAsAtomicUnit=on
  TQ_R : Outport
  TQ_L : Outport  Port=2
  TT : Outport  Port=3
  wires:
  AP/1 -> Torque demanded by the driver/1(AP)
  pedal_sat_down/1 -> Torque demanded by the driver/2(pedal_sat_down)
  pedal_sat_up/1 -> Torque demanded by the driver/3(pedal_sat_up)
  max_torque/1 -> Torque demanded by the driver/4(max_torque)
  Torque demanded by the driver/1(Throttle_Torque) -> Saturation/1
  Saturation/1 -> TT/1, TQ_R/1, TQ_L/1
  max_wheel_w/1 -> Torque demanded by the driver/5(max_wheel_w)

== system VDC_2023/ACCELERATION/RIGIDAXLE ==
  note: TOTAL FAILURE: NO ELIPSE NO INVERTER SPEED
  Throttle_Torque [Nm] : Inport
  Action Port : ActionPort  ActionPortLabel=else
  "Rigid Axle 2024 " : MATLAB Function  TreatAsAtomicUnit=on
  RigidAxle : Constant  Value=4
  Tq_RR_SM4 [Nm] (0,27) : Outport  VectorParamsAs1DForOutWhenUnconnected=off
  Tq_RL_SM4 [Nm] (0,27) : Outport  Port=2  VectorParamsAs1DForOutWhenUnconnected=off
  sensorics_mode : Outport  Port=3
  wires:
  "Rigid Axle 2024 "/1(Motor_Torque_RR) -> Tq_RR_SM4 [Nm] (0,27)/1
  "Rigid Axle 2024 "/2(Motor_Torque_RL) -> Tq_RL_SM4 [Nm] (0,27)/1
  Throttle_Torque [Nm]/1 -> "Rigid Axle 2024 "/1(Throttle_Torque)
  RigidAxle/1 -> sensorics_mode/1

== system VDC_2023/ACCELERATION/RIGIDAXLE WITH TC ==
  note: ONLY ELLIPSE AND INVERTER SPEEDS
  RR_Vel_ms_Wheel [m/s] : Inport
  RL_Vel_ms_Wheel [m/s] : Inport  Port=2
  Throttle_Torque [Nm] : Inport  Port=3
  MAX_SLR : Inport  Port=4
  el_Vel_X [m/s] : Inport  Port=5
  Action Port : ActionPort  ActionPortLabel=if(u1 <= 2)
  Max : MinMax  Function=max  Inputs=2
  "Rigid Axle with TC 2024 " : MATLAB Function  TreatAsAtomicUnit=on
  RigidAxleTC : Constant  Value=2
  Tq_RR_SM2 [Nm] (0,27) : Outport  VectorParamsAs1DForOutWhenUnconnected=off
  Tq_RL_SM2 [Nm] (0,27) : Outport  Port=2  VectorParamsAs1DForOutWhenUnconnected=off
  sensorics_mode : Outport  Port=3
  wires:
  RR_Vel_ms_Wheel [m/s]/1 -> Max/1
  "Rigid Axle with TC 2024 "/1(Motor_Torque_RR) -> Tq_RR_SM2 [Nm] (0,27)/1
  "Rigid Axle with TC 2024 "/2(Motor_Torque_RL) -> Tq_RL_SM2 [Nm] (0,27)/1
  Max/1 -> "Rigid Axle with TC 2024 "/4(Max_Vel_ms_Wheel)
  RL_Vel_ms_Wheel [m/s]/1 -> Max/2
  Throttle_Torque [Nm]/1 -> "Rigid Axle with TC 2024 "/2(Throttle_Torque)
  MAX_SLR/1 -> "Rigid Axle with TC 2024 "/1(MAX_SLR)
  el_Vel_X [m/s]/1 -> "Rigid Axle with TC 2024 "/3(el_Vel_X)
  RigidAxleTC/1 -> sensorics_mode/1

== system VDC_2023/AUTOX1/RIGIDAXLE ==
  note: TOTAL FAILURE: NO ELIPSE NO INVERTER SPEED
  Throttle_Torque [Nm] : Inport
  Action Port : ActionPort  ActionPortLabel=else
  "Rigid Axle 2024 " : MATLAB Function  TreatAsAtomicUnit=on
  RigidAxle : Constant  Value=4
  Tq_RR_SM4 [Nm] (0,27) : Outport  VectorParamsAs1DForOutWhenUnconnected=off
  Tq_RL_SM4 [Nm] (0,27) : Outport  Port=2  VectorParamsAs1DForOutWhenUnconnected=off
  sensorics_mode : Outport  Port=3
  wires:
  RigidAxle/1 -> sensorics_mode/1
  Throttle_Torque [Nm]/1 -> "Rigid Axle 2024 "/1(Throttle_Torque)
  "Rigid Axle 2024 "/2(Motor_Torque_RL) -> Tq_RL_SM4 [Nm] (0,27)/1
  "Rigid Axle 2024 "/1(Motor_Torque_RR) -> Tq_RR_SM4 [Nm] (0,27)/1

== system VDC_2023/AUTOX1/RIGIDAXLE WITH TC ==
  RR_Vel_ms_Wheel [m/s] : Inport
  RL_Vel_ms_Wheel [m/s] : Inport  Port=2
  Throttle_Torque [Nm] : Inport  Port=3
  MAX_SLR : Inport  Port=4
  el_Vel_X [m/s] : Inport  Port=5
  Action Port : ActionPort  ActionPortLabel=elseif(u1 == 2)
  Max : MinMax  Function=max  Inputs=2
  "Rigid Axle with TC 2024 " : MATLAB Function  TreatAsAtomicUnit=on
  RigidAxleTC : Constant  Value=2
  Tq_RR_SM2 [Nm] (0,27) : Outport  VectorParamsAs1DForOutWhenUnconnected=off
  Tq_RL_SM2 [Nm] (0,27) : Outport  Port=2  VectorParamsAs1DForOutWhenUnconnected=off
  sensorics_mode : Outport  Port=3
  wires:
  RigidAxleTC/1 -> sensorics_mode/1
  el_Vel_X [m/s]/1 -> "Rigid Axle with TC 2024 "/3(el_Vel_X)
  MAX_SLR/1 -> "Rigid Axle with TC 2024 "/1(MAX_SLR)
  Throttle_Torque [Nm]/1 -> "Rigid Axle with TC 2024 "/2(Throttle_Torque)
  RL_Vel_ms_Wheel [m/s]/1 -> Max/2
  Max/1 -> "Rigid Axle with TC 2024 "/4(Max_Vel_ms_Wheel)
  "Rigid Axle with TC 2024 "/2(Motor_Torque_RL) -> Tq_RL_SM2 [Nm] (0,27)/1
  "Rigid Axle with TC 2024 "/1(Motor_Torque_RR) -> Tq_RR_SM2 [Nm] (0,27)/1
  RR_Vel_ms_Wheel [m/s]/1 -> Max/1

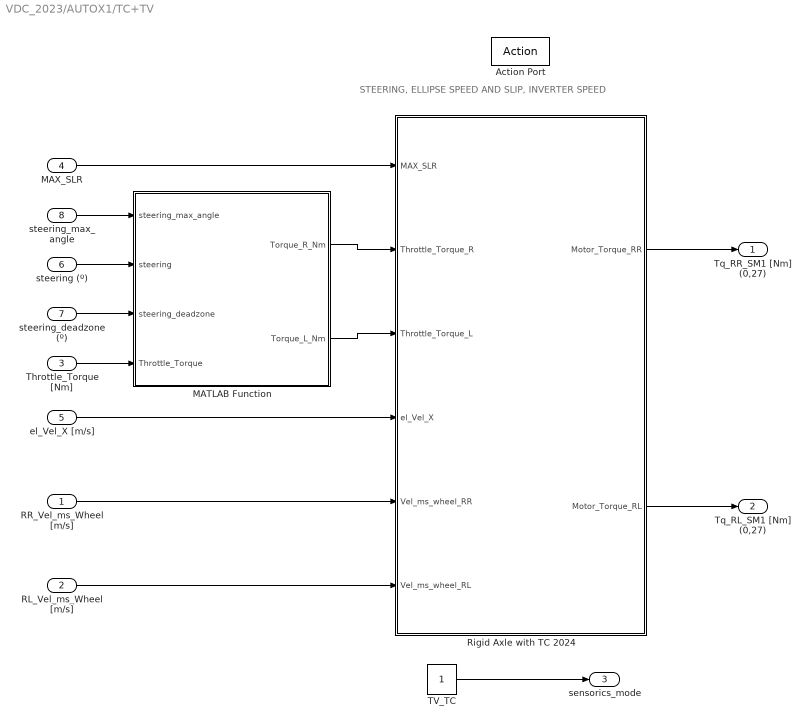
== system VDC_2023/AUTOX1/TC+TV ==
  note: STEERING, ELLIPSE SPEED AND SLIP, INVERTER SPEED
  RR_Vel_ms_Wheel [m/s] : Inport
  RL_Vel_ms_Wheel [m/s] : Inport  Port=2
  Throttle_Torque [Nm] : Inport  Port=3
  MAX_SLR : Inport  Port=4
  el_Vel_X [m/s] : Inport  Port=5
  steering (º) : Inport  Port=6
  steering_deadzone (º) : Inport  Port=7
  steering_max_angle : Inport  Port=8
  Action Port : ActionPort  ActionPortLabel=if(u1 ==1)
  MATLAB Function : MATLAB Function  TreatAsAtomicUnit=on
  "Rigid Axle with TC 2024 " : MATLAB Function  TreatAsAtomicUnit=on
  TV_TC : Constant
  Tq_RR_SM1 [Nm] (0,27) : Outport  VectorParamsAs1DForOutWhenUnconnected=off
  Tq_RL_SM1 [Nm] (0,27) : Outport  Port=2  VectorParamsAs1DForOutWhenUnconnected=off
  sensorics_mode : Outport  Port=3
  wires:
  TV_TC/1 -> sensorics_mode/1
  MATLAB Function/2(Torque_L_Nm) -> "Rigid Axle with TC 2024 "/3(Throttle_Torque_L)
  steering_max_angle/1 -> MATLAB Function/1(steering_max_angle)
  steering_deadzone (º)/1 -> MATLAB Function/3(steering_deadzone)
  steering (º)/1 -> MATLAB Function/2(steering)
  el_Vel_X [m/s]/1 -> "Rigid Axle with TC 2024 "/4(el_Vel_X)
  MAX_SLR/1 -> "Rigid Axle with TC 2024 "/1(MAX_SLR)
  MATLAB Function/1(Torque_R_Nm) -> "Rigid Axle with TC 2024 "/2(Throttle_Torque_R)
  RL_Vel_ms_Wheel [m/s]/1 -> "Rigid Axle with TC 2024 "/6(Vel_ms_wheel_RL)
  "Rigid Axle with TC 2024 "/2(Motor_Torque_RL) -> Tq_RL_SM1 [Nm] (0,27)/1
  "Rigid Axle with TC 2024 "/1(Motor_Torque_RR) -> Tq_RR_SM1 [Nm] (0,27)/1
  RR_Vel_ms_Wheel [m/s]/1 -> "Rigid Axle with TC 2024 "/5(Vel_ms_wheel_RR)
  Throttle_Torque [Nm]/1 -> MATLAB Function/4(Throttle_Torque)

== system VDC_2023/ENDURANCE/RIGIDAXLE ==
  note: TOTAL FAILURE: NO ELIPSE NO INVERTER SPEED
  Throttle_Torque [Nm] : Inport
  Action Port : ActionPort  ActionPortLabel=else
  "Rigid Axle 2024 " : MATLAB Function  TreatAsAtomicUnit=on
  RigidAxle : Constant  Value=4
  Tq_RR_SM4 [Nm] (0,27) : Outport  VectorParamsAs1DForOutWhenUnconnected=off
  Tq_RL_SM4 [Nm] (0,27) : Outport  Port=2  VectorParamsAs1DForOutWhenUnconnected=off
  sensorics_mode : Outport  Port=3
  wires:
  "Rigid Axle 2024 "/1(Motor_Torque_RR) -> Tq_RR_SM4 [Nm] (0,27)/1
  "Rigid Axle 2024 "/2(Motor_Torque_RL) -> Tq_RL_SM4 [Nm] (0,27)/1
  Throttle_Torque [Nm]/1 -> "Rigid Axle 2024 "/1(Throttle_Torque)
  RigidAxle/1 -> sensorics_mode/1

== system VDC_2023/ENDURANCE/RIGIDAXLE WITH TC ==
  note: ONLY ELLIPSE AND INVERTER SPEEDS
  RR_Vel_ms_Wheel [m/s] : Inport
  RL_Vel_ms_Wheel [m/s] : Inport  Port=2
  Throttle_Torque [Nm] : Inport  Port=3
  MAX_SLR : Inport  Port=4
  el_Vel_X [m/s] : Inport  Port=5
  Action Port : ActionPort  ActionPortLabel=elseif(u1 == 2)
  Max : MinMax  Function=max  Inputs=2
  "Rigid Axle with TC 2024 " : MATLAB Function  TreatAsAtomicUnit=on
  RigidAxleTC : Constant  Value=2
  Tq_RR_SM2 [Nm] (0,27) : Outport  VectorParamsAs1DForOutWhenUnconnected=off
  Tq_RL_SM2 [Nm] (0,27) : Outport  Port=2  VectorParamsAs1DForOutWhenUnconnected=off
  sensorics_mode : Outport  Port=3
  wires:
  RR_Vel_ms_Wheel [m/s]/1 -> Max/1
  "Rigid Axle with TC 2024 "/1(Motor_Torque_RR) -> Tq_RR_SM2 [Nm] (0,27)/1
  "Rigid Axle with TC 2024 "/2(Motor_Torque_RL) -> Tq_RL_SM2 [Nm] (0,27)/1
  Max/1 -> "Rigid Axle with TC 2024 "/4(Max_Vel_ms_Wheel)
  RL_Vel_ms_Wheel [m/s]/1 -> Max/2
  Throttle_Torque [Nm]/1 -> "Rigid Axle with TC 2024 "/2(Throttle_Torque)
  MAX_SLR/1 -> "Rigid Axle with TC 2024 "/1(MAX_SLR)
  el_Vel_X [m/s]/1 -> "Rigid Axle with TC 2024 "/3(el_Vel_X)
  RigidAxleTC/1 -> sensorics_mode/1

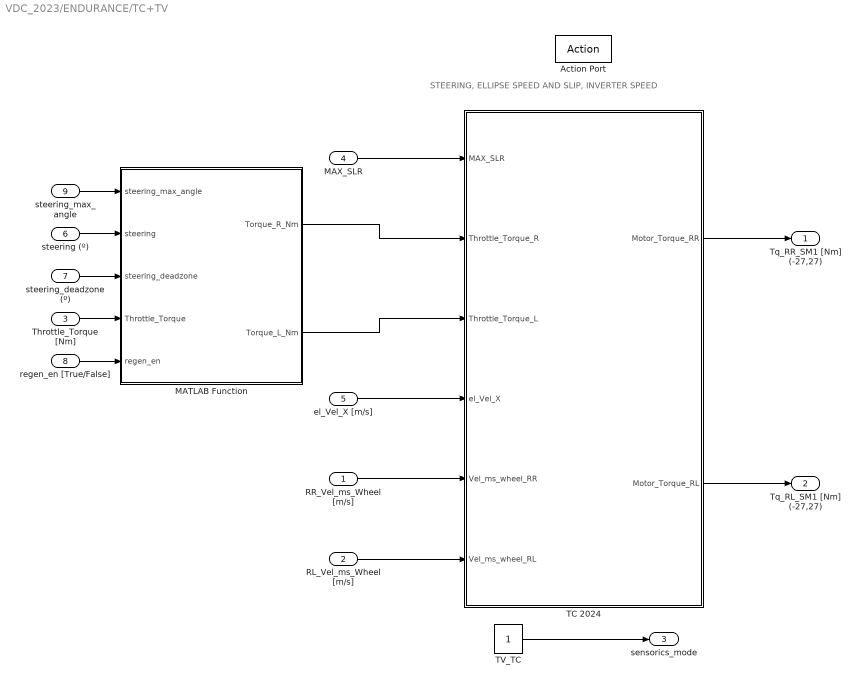
== system VDC_2023/ENDURANCE/TC+TV ==
  note: STEERING, ELLIPSE SPEED AND SLIP, INVERTER SPEED
  RR_Vel_ms_Wheel [m/s] : Inport
  RL_Vel_ms_Wheel [m/s] : Inport  Port=2
  Throttle_Torque [Nm] : Inport  Port=3
  MAX_SLR : Inport  Port=4
  el_Vel_X [m/s] : Inport  Port=5
  steering (º) : Inport  Port=6
  steering_deadzone (º) : Inport  Port=7
  regen_en [True/False] : Inport  Port=8
  steering_max_angle : Inport  Port=9
  Action Port : ActionPort  ActionPortLabel=if(u1 ==1)
  MATLAB Function : MATLAB Function  TreatAsAtomicUnit=on
  TC 2024 : MATLAB Function  TreatAsAtomicUnit=on
  TV_TC : Constant
  Tq_RR_SM1 [Nm] (-27,27) : Outport  VectorParamsAs1DForOutWhenUnconnected=off
  Tq_RL_SM1 [Nm] (-27,27) : Outport  Port=2  VectorParamsAs1DForOutWhenUnconnected=off
  sensorics_mode : Outport  Port=3
  wires:
  RR_Vel_ms_Wheel [m/s]/1 -> TC 2024/5(Vel_ms_wheel_RR)
  TC 2024/1(Motor_Torque_RR) -> Tq_RR_SM1 [Nm] (-27,27)/1
  TC 2024/2(Motor_Torque_RL) -> Tq_RL_SM1 [Nm] (-27,27)/1
  RL_Vel_ms_Wheel [m/s]/1 -> TC 2024/6(Vel_ms_wheel_RL)
  Throttle_Torque [Nm]/1 -> MATLAB Function/4(Throttle_Torque)
  MATLAB Function/1(Torque_R_Nm) -> TC 2024/2(Throttle_Torque_R)
  MAX_SLR/1 -> TC 2024/1(MAX_SLR)
  el_Vel_X [m/s]/1 -> TC 2024/4(el_Vel_X)
  steering (º)/1 -> MATLAB Function/2(steering)
  steering_deadzone (º)/1 -> MATLAB Function/3(steering_deadzone)
  regen_en [True/False]/1 -> MATLAB Function/5(regen_en)
  steering_max_angle/1 -> MATLAB Function/1(steering_max_angle)
  MATLAB Function/2(Torque_L_Nm) -> TC 2024/3(Throttle_Torque_L)
  TV_TC/1 -> sensorics_mode/1

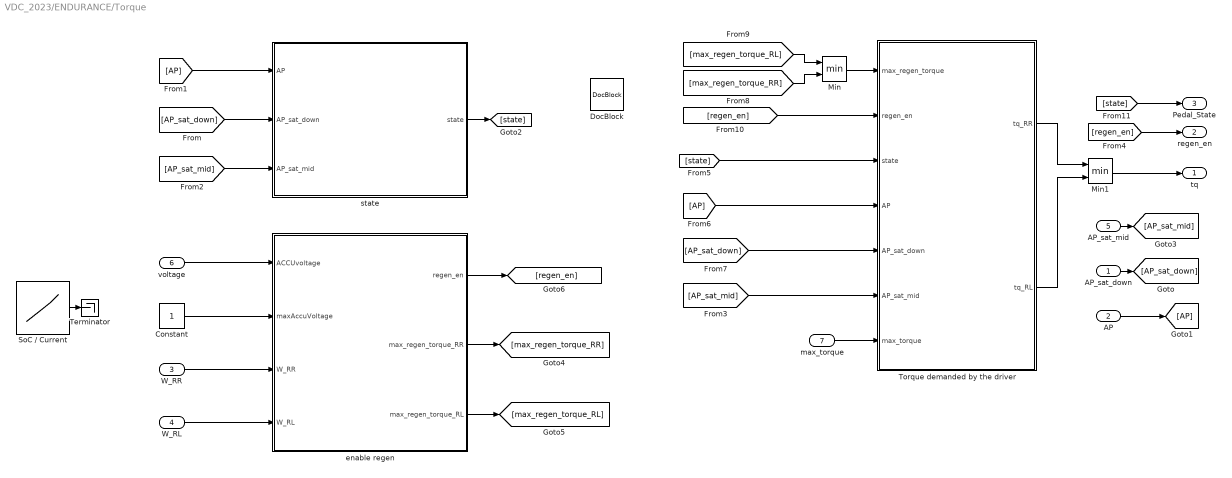
== system VDC_2023/ENDURANCE/Torque ==
  AP_sat_down : Inport
  AP : Inport  Port=2
  W_RR : Inport  Port=3
  W_RL : Inport  Port=4
  AP_sat_mid : Inport  Port=5
  voltage : Inport  Port=6
  max_torque : Inport  Port=7
  Constant : Constant
  DocBlock : simulink/Model-Wide Utilities/DocBlock  DocumentType=Text
      content=|
      | FUNCIONAMENT DEL SUBSISTEMA
      | per especificacions d'accu, hem de implementar un "lift and coast" per a maximitzar la duració
      | de l'accu i intentar completar la endurance.
      | Per a fer això, s'ha decidit dividir el pedal en 3 zones. Parlarem del recorregut de 0 a 1,
      | sent 0=0º i 1=30º: de 0 a 0.4 el cotxe farà regenerativa, de 0.4 a 0.5 el motor no aplicarà cap força
      | i de 0.5 a 1 el motor accelera el monoplaça.
      |
      | El bloc state determina a quin punt del recorregut del accelerador estem.
      | El bloc regen calcula el torque màxim de frenada que podem aplicar.
      | El bloc torque calcula el torque a aplicar segons l'estat del pedal i els torques de regen.
  Min : MinMax  Inputs=2
  Min1 : MinMax  Inputs=2
  SoC / Current : Lookup_n-D  NumberOfTableDimensions=1  BreakpointsForDimension1=[0.5;0.625;0.75;0.875;1;1.125;1.25;1.375;1.5;1.625;1.75;1.875;2;2.125;2.25;2.375;2.5;2.625;2.75;2.875;3;3.125;3.25;3.375;3.5;3.625;3.75;3.875;4;4.125;4.25;4.375;4.5;4.625;4.75;4.875;5;5.125;5.25;5.375;5.5;5.625;5.75;5.875;6;6.125;6.25;6.375;6.5;6.625;6.75;6.875;7;7.125;7.25;7.375;7.5;7.625;7.75;7.875;8;8.125;8.25;8.375;8.5;8.625;8.75;8.875;9;9.125;9.25;9.375;9.5;9.625;9.75;9.875;10;10.125;10.25;10.375;10.5;10.625;10.75;10.875;11;11.125;11.25;11.375;11.5;11.625;11.75;11.875;12;12.125;12.25;12.375;12.5;12.625;12.75;12.875;13;13.125;13.25;13.375;13.5;13.625;13.75;13.875;14;14.125;14.25;14.375;14.5;14.625;14.75;14.875;15;15.125;15.25;15.375;15.5;15.625;15.75;15.875;16;16.125;16.25;16.375;16.5;16.625;16.75;16.875;17;17.125;17.25;17.375;17.5;17.625;17.75;17.875;18;18.125;18.25;18.375;18.5;18.625;18.75;18.875;19;19.125;19.25;19.375;19.5;19.625;19.75;19.875;20]  Table=[99.8638515373959;99.8261032164556;99.787078895957;99.7464496412943;99.7031623399186;99.6569399822743;99.6085457240994;99.5583542992092;99.5063175156323;99.4531242547042;99.3996199106189;99.3457555385114;99.2916196918623;99.236840468825;99.1815776579033;99.1261581819638;99.0704600282389;99.0145621384686;98.9579862041378;98.9007649443125;98.8435709856118;98.7866964363398;98.7294309904695;98.6720632124312;98.6150692116673;98.5583262081729;98.5016459402354;98.4450485815784;98.3886324537531;98.3323113111552;98.2760370231491;98.219889318764;98.1640621452933;98.1086506246766;98.0534368997348;97.9982819285613;97.9430609511937;97.8873777779768;97.8316006765195;97.7756093847174;97.7196164319235;97.6636145234219;97.6074949919914;97.5512806941619;97.4949079148039;97.4386383393529;97.3824957659839;97.3265205156682;97.2707949766523;97.2152161070864;97.1597722415201;97.1042534409084;97.0487976906826;96.9934428687166;96.9382597426796;96.8831834289612;96.8282192088546;96.7734442056342;96.7189107658621;96.6645220082209;96.6101480019029;96.5557548375112;96.5011588175642;96.4465366275317;96.3919193515209;96.3373265852361;96.2827271967385;96.2284708305744;96.1743003814294;96.1202272122311;96.0662507872358;96.0124620565115;95.9587960858038;95.9054190254676;95.8523021379409;95.7996353499439;95.7473738162933;95.6954428515415;95.6440855591069;95.5931379659417;95.542675825155;95.4925898155832;95.4427621694762;95.3932593338181;95.3439201852395;95.2945061423096;95.2453155323362;95.1967449588083;95.1483471741501;95.1006171187692;95.05309426103;95.0060982834647;94.9596397012176;94.9136340068524;94.8681131899029;94.8228748176359;94.7773623572551;94.7323289961706;94.6877507845258;94.6438926674393;94.6005330360533;94.5579519678426;94.5157187867765;94.4736889382833;94.4318130425109;94.3900803949631;94.3486100596819;94.3072893708641;94.2662109590131;94.2257873041514;94.1857638071793;94.1462094608166;94.1070508764276;94.0683633537351;94.0297036137025;93.991181303978;93.9530103965701;93.9150714405644;93.8775886864698;93.840470618768;93.8039440022059;93.7678066751737;93.732300190504;93.6974844310299;93.6632820753455;93.6298210766945;93.5968199450375;93.5642570674136;93.5321287740758;93.5005594977202;93.4694689466742;93.4389330496507;93.4087179396065;93.3791648078586;93.3504222584188;93.3220395833837;93.2930881546744;93.2647696405904;93.2369762454977;93.2098304380767;93.1829890047197;93.156614414508;93.1307021213018;93.1049104059305;93.0794093899284;93.0544610934045;93.0299137147753;93.0061930132338;92.9829950868456;92.9601547660346;92.9377957962841;92.9158579087248;92.8941701658703;92.8727117435597;92.851501872486;92.8305232504108;92.8100674242247]  InternalRulePriority=Speed  RndMeth=Simplest
  Terminator : Terminator
  Torque demanded by the driver : MATLAB Function  TreatAsAtomicUnit=on
  enable regen : MATLAB Function  TreatAsAtomicUnit=on
  state : MATLAB Function  TreatAsAtomicUnit=on
  tq : Outport
  regen_en : Outport  Port=2
  Pedal_State : Outport  Port=3
  wires:
  W_RR/1 -> enable regen/3(W_RR)
  W_RL/1 -> enable regen/4(W_RL)
  AP_sat_down/1 -> [AP_sat_down]
  [AP_sat_down] -> state/2(AP_sat_down)
  AP/1 -> [AP]
  [AP] -> state/1(AP)
  [AP] -> Torque demanded by the driver/4(AP)
  [AP_sat_down] -> Torque demanded by the driver/5(AP_sat_down)
  enable regen/2(max_regen_torque_RR) -> [max_regen_torque_RR]
  enable regen/3(max_regen_torque_RL) -> [max_regen_torque_RL]
  enable regen/1(regen_en) -> [regen_en]
  [regen_en] -> Torque demanded by the driver/2(regen_en)
  state/1(state) -> [state]
  [max_regen_torque_RR] -> Min/2
  [max_regen_torque_RL] -> Min/1
  Min/1 -> Torque demanded by the driver/1(max_regen_torque)
  AP_sat_mid/1 -> [AP_sat_mid]
  [AP_sat_mid] -> state/3(AP_sat_mid)
  [AP_sat_mid] -> Torque demanded by the driver/6(AP_sat_mid)
  Torque demanded by the driver/1(tq_RR) -> Min1/1
  Torque demanded by the driver/2(tq_RL) -> Min1/2
  Min1/1 -> tq/1
  [regen_en] -> regen_en/1
  voltage/1 -> enable regen/1(ACCUvoltage)
  [state] -> Torque demanded by the driver/3(state)
  [state] -> Pedal_State/1
  max_torque/1 -> Torque demanded by the driver/7(max_torque)
  SoC / Current/1 -> Terminator/1
  Constant/1 -> enable regen/2(maxAccuVoltage)

== system VDC_2023/ENDURANCE/Velocity cap ==
  Tq_RR : Inport
  Tq_RL : Inport  Port=2
  V_CG : Inport  Port=3
  If : If  IfExpression=u1 > 15
  If Action Subsystem : Subsystem  TreatAsAtomicUnit=on
  If Action Subsystem1 : Subsystem  TreatAsAtomicUnit=on
  Merge : Merge
  Merge1 : Merge
  TQ_RR : Outport
  TQ_RL : Outport  Port=2
  wires:
  V_CG/1 -> If/1
  Tq_RR/1 -> If Action Subsystem1/1(Tq_RR), If Action Subsystem/1(Tq_RR)
  Tq_RL/1 -> If Action Subsystem1/2(Tq_RL), If Action Subsystem/2(Tq_RL)
  If Action Subsystem/2(TQ_RL) -> Merge/1
  If Action Subsystem1/1(TQ_RL) -> Merge/2
  Merge/1 -> TQ_RL/1
  If Action Subsystem/1(TQ_RR) -> Merge1/1
  If Action Subsystem1/2(TQ_RR) -> Merge1/2
  Merge1/1 -> TQ_RR/1
  If/2 -> If Action Subsystem1/Action
  If/1 -> If Action Subsystem/Action

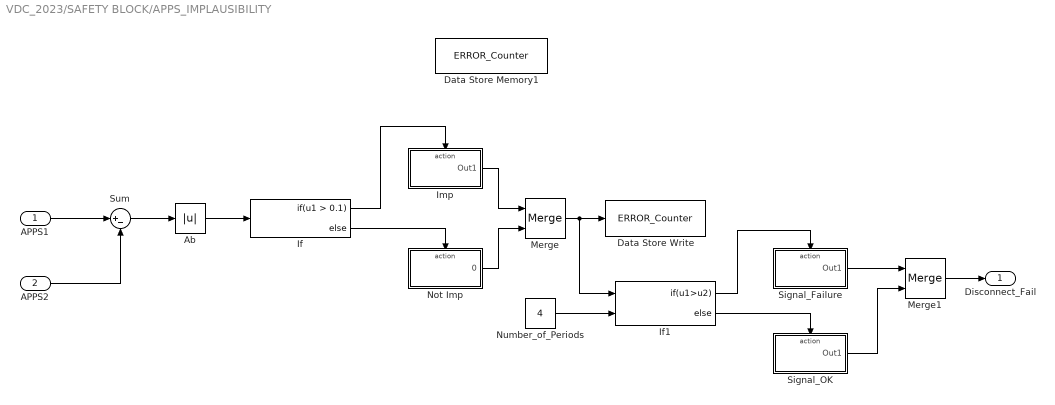
== system VDC_2023/SAFETY BLOCK/APPS_IMPLAUSIBILITY ==
  APPS1 : Inport
  APPS2 : Inport  Port=2
  Ab : Abs  SaturateOnIntegerOverflow=off
  Data Store Memory1 : DataStoreMemory  DataStoreName=ERROR_Counter  ReadBeforeWriteMsg=warning  WriteAfterWriteMsg=warning  WriteAfterReadMsg=warning  ShowAdditionalParam=off
  Data Store Write : DataStoreWrite  DataStoreName=ERROR_Counter  IndexOptions=Index vector (dialog)  Indices=1  OutputSizes=1
  If : If  IfExpression=u1 > 0.1
  If1 : If  NumInputs=2  IfExpression=u1>u2
  Imp : Subsystem  TreatAsAtomicUnit=on
  Merge : Merge
  Merge1 : Merge
  Not Imp : Subsystem  TreatAsAtomicUnit=on
  Number_of_Periods : Constant  Value=4
  Signal_Failure : Subsystem  TreatAsAtomicUnit=on
  Signal_OK : Subsystem  TreatAsAtomicUnit=on
  Sum : Sum  Inputs=|+-
  Disconnect_Fail : Outport  VectorParamsAs1DForOutWhenUnconnected=off
  wires:
  Number_of_Periods/1 -> If1/2
  Imp/1(Out1) -> Merge/1
  Signal_Failure/1(Out1) -> Merge1/1
  Signal_OK/1(Out1) -> Merge1/2
  Merge1/1 -> Disconnect_Fail/1
  APPS1/1 -> Sum/1
  If/1 -> Imp/Action
  If1/2 -> Signal_OK/Action
  Merge/1 -> Data Store Write/1, If1/1
  If1/1 -> Signal_Failure/Action
  APPS2/1 -> Sum/2
  Ab/1 -> If/1
  If/2 -> Not Imp/Action
  Sum/1 -> Ab/1
  Not Imp/1(0) -> Merge/2

== system VDC_2023/SKIDPAD/RIGIDAXLE ==
  note: TOTAL FAILURE: NO ELIPSE NO INVERTER SPEED
  Throttle_Torque [Nm] : Inport
  Action Port : ActionPort  ActionPortLabel=else
  "Rigid Axle 2024 " : MATLAB Function  TreatAsAtomicUnit=on
  RigidAxle : Constant  Value=4
  Tq_RR_SM4 [Nm] (0,27) : Outport  VectorParamsAs1DForOutWhenUnconnected=off
  Tq_RL_SM4 [Nm] (0,27) : Outport  Port=2  VectorParamsAs1DForOutWhenUnconnected=off
  sensorics_mode : Outport  Port=3
  wires:
  "Rigid Axle 2024 "/1(Motor_Torque_RR) -> Tq_RR_SM4 [Nm] (0,27)/1
  "Rigid Axle 2024 "/2(Motor_Torque_RL) -> Tq_RL_SM4 [Nm] (0,27)/1
  Throttle_Torque [Nm]/1 -> "Rigid Axle 2024 "/1(Throttle_Torque)
  RigidAxle/1 -> sensorics_mode/1

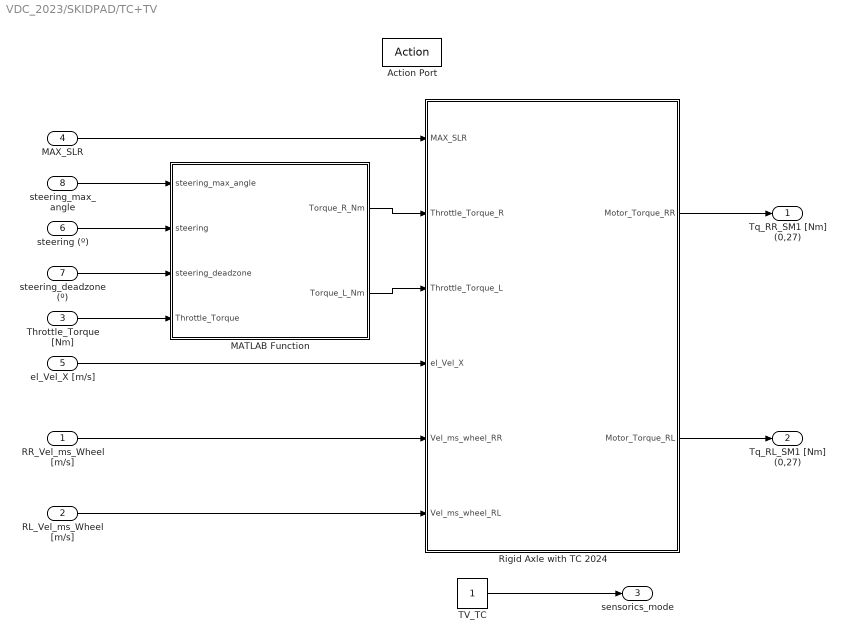
== system VDC_2023/SKIDPAD/TC+TV ==
  RR_Vel_ms_Wheel [m/s] : Inport
  RL_Vel_ms_Wheel [m/s] : Inport  Port=2
  Throttle_Torque [Nm] : Inport  Port=3
  MAX_SLR : Inport  Port=4
  el_Vel_X [m/s] : Inport  Port=5
  steering (º) : Inport  Port=6
  steering_deadzone (º) : Inport  Port=7
  steering_max_angle : Inport  Port=8
  Action Port : ActionPort  ActionPortLabel=if(u1 == 1)
  MATLAB Function : MATLAB Function  TreatAsAtomicUnit=on
  "Rigid Axle with TC 2024 " : MATLAB Function  TreatAsAtomicUnit=on
  TV_TC : Constant
  Tq_RR_SM1 [Nm] (0,27) : Outport  VectorParamsAs1DForOutWhenUnconnected=off
  Tq_RL_SM1 [Nm] (0,27) : Outport  Port=2  VectorParamsAs1DForOutWhenUnconnected=off
  sensorics_mode : Outport  Port=3
  wires:
  RR_Vel_ms_Wheel [m/s]/1 -> "Rigid Axle with TC 2024 "/5(Vel_ms_wheel_RR)
  "Rigid Axle with TC 2024 "/1(Motor_Torque_RR) -> Tq_RR_SM1 [Nm] (0,27)/1
  "Rigid Axle with TC 2024 "/2(Motor_Torque_RL) -> Tq_RL_SM1 [Nm] (0,27)/1
  RL_Vel_ms_Wheel [m/s]/1 -> "Rigid Axle with TC 2024 "/6(Vel_ms_wheel_RL)
  Throttle_Torque [Nm]/1 -> MATLAB Function/4(Throttle_Torque)
  MATLAB Function/1(Torque_R_Nm) -> "Rigid Axle with TC 2024 "/2(Throttle_Torque_R)
  MAX_SLR/1 -> "Rigid Axle with TC 2024 "/1(MAX_SLR)
  el_Vel_X [m/s]/1 -> "Rigid Axle with TC 2024 "/4(el_Vel_X)
  steering (º)/1 -> MATLAB Function/2(steering)
  steering_deadzone (º)/1 -> MATLAB Function/3(steering_deadzone)
  steering_max_angle/1 -> MATLAB Function/1(steering_max_angle)
  MATLAB Function/2(Torque_L_Nm) -> "Rigid Axle with TC 2024 "/3(Throttle_Torque_L)
  TV_TC/1 -> sensorics_mode/1

== system VDC_2023/SKIDPAD/TV with TC OFF  ==
  Throttle_Torque [Nm] : Inport
  steering_deadzone : Inport  Port=2
  steering : Inport  Port=3
  steering_max_angle : Inport  Port=4
  Action Port : ActionPort  ActionPortLabel=elseif(u1 <= 3)
  MATLAB Function : MATLAB Function  TreatAsAtomicUnit=on
  SteeringTV : Constant  Value=3
  Tq_RR_SM3 [Nm] (0,27) : Outport  VectorParamsAs1DForOutWhenUnconnected=off
  Tq_RL_SM3 [Nm] (0,27) : Outport  Port=2  VectorParamsAs1DForOutWhenUnconnected=off
  sensorics_mode : Outport  Port=3
  wires:
  Throttle_Torque [Nm]/1 -> MATLAB Function/4(Throttle_Torque)
  steering_deadzone/1 -> MATLAB Function/3(steering_deadzone)
  steering/1 -> MATLAB Function/2(steering)
  steering_max_angle/1 -> MATLAB Function/1(steering_max_angle)
  MATLAB Function/1(Torque_R_Nm) -> Tq_RR_SM3 [Nm] (0,27)/1
  MATLAB Function/2(Torque_L_Nm) -> Tq_RL_SM3 [Nm] (0,27)/1
  SteeringTV/1 -> sensorics_mode/1

== system VDC_2023/TEST_MODE_IN/BYPASS ==
  In1 : Inport
  In2 : Inport  Port=2
  In3 : Inport  Port=3
  In4 : Inport  Port=4
  Action Port : ActionPort  ActionPortLabel=else
  Out1 : Outport  VectorParamsAs1DForOutWhenUnconnected=off
  Out2 : Outport  Port=2  VectorParamsAs1DForOutWhenUnconnected=off
  Out3 : Outport  Port=3  VectorParamsAs1DForOutWhenUnconnected=off
  Out4 : Outport  Port=4  VectorParamsAs1DForOutWhenUnconnected=off
  wires:
  In1/1 -> Out1/1
  In2/1 -> Out2/1
  In3/1 -> Out3/1
  In4/1 -> Out4/1

== system VDC_2023/TEST_MODE_IN/TEST_CONSTANTS ==
  Action Port : ActionPort  ActionPortLabel=if(u1 == 1)
  Constant{,1..3} (4 alike) : Constant  Value=800
  Out1 : Outport  VectorParamsAs1DForOutWhenUnconnected=off
  Out2 : Outport  Port=2  VectorParamsAs1DForOutWhenUnconnected=off
  Out3 : Outport  Port=3  VectorParamsAs1DForOutWhenUnconnected=off
  Out4 : Outport  Port=4  VectorParamsAs1DForOutWhenUnconnected=off
  wires:
  Constant/1 -> Out1/1
  Constant1/1 -> Out2/1
  Constant2/1 -> Out3/1
  Constant3/1 -> Out4/1

== system VDC_2023/ENDURANCE/Velocity cap/If Action Subsystem ==
  Tq_RR : Inport
  Tq_RL : Inport  Port=2
  Action Port : ActionPort  ActionPortLabel=if(u1 > 15)
  Gain : Gain  Gain=0.25
  Gain1 : Gain  Gain=0.25
  TQ_RR : Outport
  TQ_RL : Outport  Port=2
  wires:
  Tq_RL/1 -> Gain1/1
  Gain1/1 -> TQ_RL/1
  Tq_RR/1 -> Gain/1
  Gain/1 -> TQ_RR/1

== system VDC_2023/ENDURANCE/Velocity cap/If Action Subsystem1 ==
  Tq_RR : Inport
  Tq_RL : Inport  Port=2
  Action Port : ActionPort  ActionPortLabel=else
  TQ_RL : Outport
  TQ_RR : Outport  Port=2
  wires:
  Tq_RR/1 -> TQ_RR/1
  Tq_RL/1 -> TQ_RL/1

== system VDC_2023/SAFETY BLOCK/APPS_IMPLAUSIBILITY/Imp ==
  Action Port : ActionPort  ActionPortLabel=if(u1 > 0.1)
  Add : Sum
  Constant : Constant  OutDataTypeStr=boolean
  Data Store Read : DataStoreRead  DataStoreName=ERROR_Counter  IndexOptions=Index vector (dialog)  Indices=1  OutputSizes=1
  Out1 : Outport  VectorParamsAs1DForOutWhenUnconnected=off
  wires:
  Data Store Read/1 -> Add/1
  Constant/1 -> Add/2
  Add/1 -> Out1/1

== system VDC_2023/SAFETY BLOCK/APPS_IMPLAUSIBILITY/Not Imp ==
  Action Port : ActionPort  ActionPortLabel=else
  Constant : Constant  Value=0  OutDataTypeStr=double
  0 : Outport  VectorParamsAs1DForOutWhenUnconnected=off
  wires:
  Constant/1 -> 0/1  "Boolean"

== system VDC_2023/SAFETY BLOCK/APPS_IMPLAUSIBILITY/Signal_Failure ==
  Action Port : ActionPort  ActionPortLabel=if(u1>u2)
  Constant : Constant
  Out1 : Outport  VectorParamsAs1DForOutWhenUnconnected=off
  wires:
  Constant/1 -> Out1/1

== system VDC_2023/SAFETY BLOCK/APPS_IMPLAUSIBILITY/Signal_OK ==
  Action Port : ActionPort  ActionPortLabel=else
  Constant : Constant  Value=0
  Out1 : Outport  VectorParamsAs1DForOutWhenUnconnected=off
  wires:
  Constant/1 -> Out1/1

== matlab function VDC_2023/Brake_Light ==
  data: BP input; RM input; BL output; PS input; BL_threshold input
function BL = Brake_Light(BP, RM, PS, BL_threshold)
% PS = 0 -> braking
% PS = 1 -> lift
% PS = 2 -> accelerating
% BL_threshold -> BrakePedal percentage to activate BrakeLight
    if ((RM == 5 && PS == 0) || (BP > BL_threshold))
        BL = 1;
        return;
    else
        BL = 0;
        return;
    end
end

== matlab function VDC_2023/Safety ==
  data: Tq_R input; Tq_OK input; Tq_L input; Torque_R output; Torque_L output; W_mot_RR input; W_mot_RL input
function [Torque_R,Torque_L]  = Safety(Tq_R, Tq_OK, Tq_L, W_mot_RR, W_mot_RL)
    if Tq_OK == 1 && (max(W_mot_RR, W_mot_RL) < (16500 * (2*pi)/60))
        Torque_R = Tq_R;
        Torque_L = Tq_L;
        return;
    else
        Torque_R = 0;
        Torque_L = 0;
        return;
    end
end
